simulink model "Copy_of_minimal_rcu_full"  (R2014b)
settings: Solver=ode4  SolverMode=SingleTasking  StartTime=0.0  StopTime=t_sim  FixedStep=sample_time_model  RelTol=1e-3
PreLoadFcn:
  | initModell
InitFcn:
  | initModell
undefined symbols (not defined in the file): FILTER_TAU_EXT, FIXED_FILTER_BANDWIDTH, FIXED_FILTER_BANDWIDTH_OBSERVER, iter, K_INV, KI2TAU_VEC, KS_trq, KT_trq, load_inertia, load_mass, MAX_CURRENT, MIN_SING_VALUE_M_CART, q0, rCEE_i, sample_time_model, sample_time_robot, tau_max
libraries: simulink x69, robotics x15, beasty_sfcns x7, lwr_dynamics x6, trafo3dLib x4, holgersRobLib x3, dspmtrx3 x1, dspinverses x1
(part 1 of 4)
settings Model: ExtModeAutoUpdateStatusClock=off  Creator=krie_ka  LastModifiedBy=lilge
settings DataIOCC: ExternalInput=[t u]  SignalLoggingSaveFormat=ModelDataLogs
settings OptimizationCC: ExpressionDepthLimit=2147483647  InitFltsAndDblsToZero=on
settings DebuggingCC: SaveWithParameterizedLinksMsg=none  UnderspecifiedInitializationDetection=Classic  MergeDetectMultiDrivingBlocksExec=none  FcnCallInpInsideContextMsg=UseLocalSettings  StateNameClashWarn=warning
settings HardwareCC: TargetHWDeviceType=32-bit Generic
settings SFSimCC: SimParseCustomCode=off
settings GRTTargetCC: TargetFcnLib=ansi_tfl_tmw.mat  CombineOutputUpdateFcns=off  GRTInterface=on

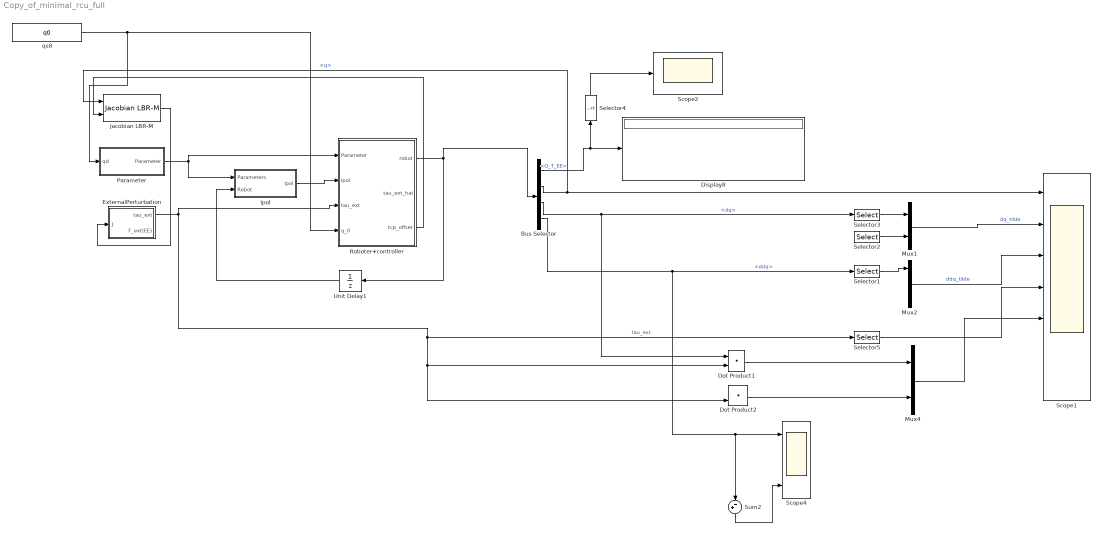
== system Copy_of_minimal_rcu_full ==
  Bus Selector : BusSelector  OutputSignals=Transform_theta.O_T_EE,q,dq,ddq
  Display8 : Display
  Dot Product1 : DotProduct  InputSameDT=on  OutDataTypeStr=Inherit: Inherit via internal rule
  Dot Product2 : DotProduct  InputSameDT=on  OutDataTypeStr=Inherit: Inherit via internal rule
  ExternalPerturbation : Subsystem
  Ipol : Subsystem
  Jacobian LBR-M : holgersRobLib/Jacobian LBR-M
  Mux1 : Mux  Inputs=2
  Mux2 : Mux  Inputs=3
  Mux4 : Mux  Inputs=2
  Parameter : Subsystem
  Roboter+controller : Subsystem
  Scope1 : Scope  NumInputPorts=7
      settings: TimeRange=1  YMin=-2~-0.04~-40~-1~-1~-1~-1  YMax=1~0.04~20~1~1~1~1  SaveName=ScopeData4
  Scope2 : Scope
      settings: TimeRange=1.4  YMin=-0.6  YMax=0.8  SaveName=ScopeData5
  Scope4 : Scope  NumInputPorts=3
      settings: TimeRange=0.06  YMin=-60~-60~-60  YMax=80~60~60  SaveName=ScopeData7
  Selector1 : Selector  InputPortWidth=7  Indices=[1:7]
  Selector2 : Selector  InputPortWidth=7  Indices=[6,7]
  Selector3 : Selector  InputPortWidth=7  Indices=[6,7]
  Selector4 : Selector  NumberOfDimensions=2  InputPortWidth=7  IndexOptions=Index vector (dialog),Index vector (dialog)  Indices=1:3,4  OutputSizes=1,1
  Selector5 : Selector  InputPortWidth=7  Indices=7
  Sum2 : Sum  Inputs=+-|
  Unit Delay1 : UnitDelay  SampleTime=-1
  qs8 : Constant  Value=q0
  wires:
  Parameter/1(Parameter) -> Roboter+controller/1(Parameter), Ipol/1(Parameters)
  Ipol/1(ipol) -> Roboter+controller/2(ipol)
  Unit Delay1/1 -> Ipol/2(Robot)
  Roboter+controller/1(robot) -> Unit Delay1/1, Bus Selector/1
  Bus Selector/3 -> Dot Product1/1, Selector3/1  "<dq>"
  Mux2/1 -> Scope1/3  "ddq_tilde"
  Bus Selector/2 -> Scope1/1, Jacobian LBR-M/1  "<q>"
  Bus Selector/1 -> Display8/1, Selector4/1  "<O_T_EE>"
  Selector1/1 -> Mux2/1
  Mux1/1 -> Scope1/2  "dq_tilde"
  Selector2/1 -> Mux1/2
  Selector3/1 -> Mux1/1
  Selector4/1 -> Scope2/1
  qs8/1 -> Parameter/1(qd), Roboter+controller/4(q_0)
  ExternalPerturbation/1(tau_ext) -> Roboter+controller/3(tau_ext), Dot Product2/2, Dot Product1/2, Selector5/1  "tau_ext"
  Selector5/1 -> Scope1/4
  Dot Product1/1 -> Mux4/1
  Dot Product2/1 -> Mux4/2
  Mux4/1 -> Scope1/5
  Jacobian LBR-M/1 -> ExternalPerturbation/1(J)
  Sum2/1 -> Scope4/3
  Bus Selector/4 -> Scope4/1, Sum2/2, Selector1/1  "<ddq>"
  Roboter+controller/3(tcp_offset) -> Jacobian LBR-M/2

== system Copy_of_minimal_rcu_full/ExternalPerturbation ==
  J : Inport
  F_ext (EE) : Constant  Tag=Fext  Value=[0; 0; 0; 0; 0; 0]
  Product : Product  Multiplication=Matrix(*)  RndMeth=Zero
  Transpose : dspmtrx3/Transpose  Hermitian=off  overflowFlag=off
  tau_ext : Outport
  F_ext(EE) : Outport  Port=2
  wires:
  Product/1 -> tau_ext/1
  J/1 -> Transpose/1
  Transpose/1 -> Product/1
  F_ext (EE)/1 -> F_ext(EE)/1, Product/2

== system Copy_of_minimal_rcu_full/Ipol ==
  Parameters : Inport
  Robot : Inport  Port=2
  Bus Creator : BusCreator  Inputs=6
  Bus Creator1 : BusCreator  Inputs=6
  Manual Switch : ManualSwitch  CurrentSetting=0
  custom : Subsystem
  dq_max1 : Constant  Value=zeros(7,1)
  dq_max5 : Constant  Value=zeros(7,1)
  dq_max6 : Constant
  dq_max7 : Constant  Value=0
  joint_ipol_5th_traj_scaling : Subsystem
  ipol : Outport
  wires:
  Parameters/1 -> custom/1(parameters), joint_ipol_5th_traj_scaling/1(parameters)
  Robot/1 -> joint_ipol_5th_traj_scaling/2(robot)
  joint_ipol_5th_traj_scaling/1(q_d) -> Bus Creator/1  "theta_d"
  joint_ipol_5th_traj_scaling/2(dq_d) -> Bus Creator/2  "dtheta_d"
  joint_ipol_5th_traj_scaling/3(ddq_d) -> Bus Creator/3  "ddtheta_d"
  joint_ipol_5th_traj_scaling/4(T_d) -> Bus Creator/4  "0_T_EE_d"
  joint_ipol_5th_traj_scaling/5(0_dX_d) -> Bus Creator/5  "0_dx_d"
  dq_max5/1 -> Bus Creator/6  "0_ddx_d"
  Bus Creator/1 -> Manual Switch/1
  dq_max6/1 -> joint_ipol_5th_traj_scaling/4(enable), joint_ipol_5th_traj_scaling/3(start1)
  dq_max7/1 -> joint_ipol_5th_traj_scaling/5(reset)
  custom/1(q_d) -> Bus Creator1/1  "theta_d"
  custom/2(dq_d) -> Bus Creator1/2  "dtheta_d"
  custom/3(ddq_d) -> Bus Creator1/3  "ddtheta_d"
  custom/4(T_d) -> Bus Creator1/4  "0_T_EE_d"
  custom/5(0_dX_d) -> Bus Creator1/5  "0_dx_d"
  dq_max1/1 -> Bus Creator1/6  "0_ddx_d"
  Bus Creator1/1 -> Manual Switch/2
  Manual Switch/1 -> ipol/1

== system Copy_of_minimal_rcu_full/Parameter ==
  qd : Inport
  Bus Creator : BusCreator  Inputs=25
  control : Subsystem
  ipol : Subsystem
  load : Subsystem
  Parameter : Outport
  wires:
  load/3(I_EE_) -> Bus Creator/3  "I_EE"
  Bus Creator/1 -> Parameter/1
  load/4(g_) -> Bus Creator/4  "g"
  control/1(controller) -> Bus Creator/5  "controller"
  control/2(enable_ffwd_vel_) -> Bus Creator/6  "enable_ffwd_vel"
  control/3(enable_ffwd_acc_) -> Bus Creator/7  "enable_ffwd_acc"
  control/4(K_theta_) -> Bus Creator/8  "K_theta"
  control/5(D_theta_) -> Bus Creator/9  "D_theta"
  control/6(TCP_T_EE_) -> Bus Creator/10  "TCP_T_EE"
  control/7(W_T_O_) -> Bus Creator/11  "W_T_0"
  control/8(EE_T_K_) -> Bus Creator/12  "EE_T_K"
  control/9(K_x_) -> Bus Creator/13  "K_x"
  control/10(D_x_) -> Bus Creator/14  "D_x"
  control/11(K_NS_) -> Bus Creator/15  "K_NS"
  control/12(Xi_NS_) -> Bus Creator/16  "Xi_NS"
  control/13(W_NS_dir_) -> Bus Creator/17  "W_NS_dir"
  load/1(m_EE_) -> Bus Creator/1  "mEE"
  load/2(rC_EE_) -> Bus Creator/2  "rC_EE"
  ipol/1(ipol_type) -> Bus Creator/18  "ipol_type"
  ipol/2(enable1) -> Bus Creator/19  "ipol_start"
  ipol/3(q2_) -> Bus Creator/20  "q2"
  ipol/4(dq_max_) -> Bus Creator/21  "dq_max"
  ipol/5(ddqd_max_) -> Bus Creator/22  "ddq_max"
  ipol/6(O_T_2_) -> Bus Creator/23  "0_T_2"
  ipol/7(O_T_d_In_) -> Bus Creator/24  "0_T_d_In"
  ipol/8(dX_max_) -> Bus Creator/25  "dX_max"
  qd/1 -> ipol/1(q2)

== system Copy_of_minimal_rcu_full/Roboter+controller ==
  Parameter : Inport
  ipol : Inport  Port=2
  tau_ext : Inport  Port=3
  q_0 : Inport  Port=4
  State_Observer : Subsystem
  controller : Subsystem
  force esimation : Subsystem
  robot_simulation : Subsystem
  robot : Outport
  tau_ext_hat : Outport  Port=2
  tcp_offset : Outport  Port=3
  wires:
  controller/1(gains) -> robot_simulation/2(gains)
  robot_simulation/1(robot) -> robot/1, force esimation/1(Robot), controller/3(robot), State_Observer/1(robot_model)
  Parameter/1 -> controller/1(parameters), robot_simulation/1(parameters)
  controller/2(tau_d) -> robot_simulation/3(tau)
  ipol/1 -> controller/2(ipol)
  State_Observer/1(r_filtered) -> tau_ext_hat/1
  tau_ext/1 -> robot_simulation/4(tau_ext)
  q_0/1 -> robot_simulation/5(q_0)
  controller/3(tcp_offset) -> tcp_offset/1
  robot_simulation/2(w/o load) -> State_Observer/2(robot_model1)
  State_Observer/2(r_filtered1) -> force esimation/2(tau_ext)

== system Copy_of_minimal_rcu_full/Ipol/custom ==
  parameters : Inport
  Bus Selector3 : BusSelector  OutputSignals=q2,dq_max,ddq_max,TCP_T_EE
  Calc Fkin2 : Subsystem  SystemSampleTime=0.034
  Clock : Clock
  Discrete Derivative1 : simulink/Discrete/Discrete Derivative  gainval=1.0  ICPrevScaledInput=0.0  InputProcessing=Inherited  OutMin=[]  OutMax=[]  OutDataType=sfix(16)  OutScaling=2^-10  DoSatur=off
  Discrete Derivative2 : simulink/Discrete/Discrete Derivative  gainval=1.0  ICPrevScaledInput=0.0  InputProcessing=Inherited  OutMin=[]  OutMax=[]  OutDataType=sfix(16)  OutScaling=2^-10  DoSatur=off
  Mux3 : Mux  Inputs=1
  Reshape1 : Reshape  OutputDimensions=[3,4]
  Reshape4 : Reshape  OutputDimensions=[3,4]
  Selector : Selector  NumberOfDimensions=2  InputPortWidth=3  IndexOptions=Index vector (dialog),Index vector (dialog)  Indices=[1:3],4  OutputSizes=1,1
  Sine Wave Function : Sin  Amplitude=0.0  Frequency=3  SampleTime=0
  Trigonometric Function : Trigonometry
  qs1 : Constant  Value=q0
  qs2 : Constant  Value=q0
  q_d : Outport
  dq_d : Outport  Port=2
  ddq_d : Outport  Port=3
  T_d : Outport  Port=4
  0_dX_d : Outport  Port=5
  wires:
  Calc Fkin2/1(FKin_d2) -> Reshape4/1, Selector/1
  Mux3/1 -> Discrete Derivative2/1, q_d/1, Calc Fkin2/1(In1)
  Selector/1 -> Discrete Derivative1/1
  Discrete Derivative1/1 -> Reshape1/1  "O_dX_d"
  Reshape1/1 -> 0_dX_d/1  "O_dX_d"
  Discrete Derivative2/1 -> dq_d/1
  qs1/1 -> Mux3/1
  Clock/1 -> Trigonometric Function/1
  Trigonometric Function/1 -> ?
  parameters/1 -> Bus Selector3/1
  Bus Selector3/4 -> Calc Fkin2/2(TCP_T_EE)  "<TCP_T_EE>"
  qs2/1 -> ddq_d/1
  Reshape4/1 -> T_d/1  "T_d"

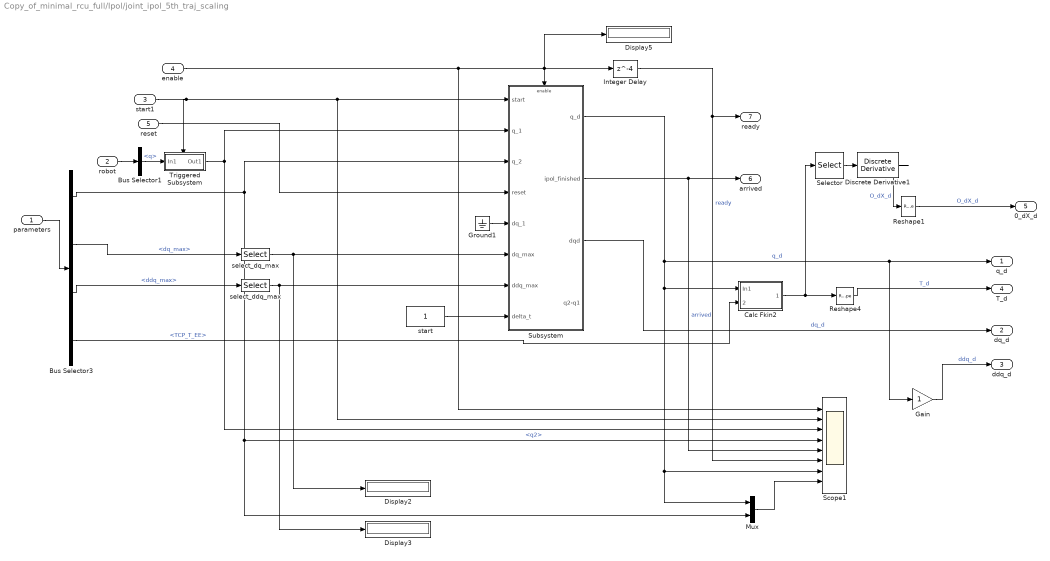
== system Copy_of_minimal_rcu_full/Ipol/joint_ipol_5th_traj_scaling ==
  parameters : Inport
  robot : Inport  Port=2
  start1 : Inport  Port=3
  enable : Inport  Port=4
  reset : Inport  Port=5
  Bus Selector1 : BusSelector  OutputSignals=q
  Bus Selector3 : BusSelector  OutputSignals=q2,dq_max,ddq_max,TCP_T_EE
  Calc Fkin2 : Subsystem  SystemSampleTime=0.034
  Discrete Derivative1 : simulink/Discrete/Discrete Derivative  gainval=1.0  ICPrevScaledInput=0.0  InputProcessing=Inherited  OutMin=[]  OutMax=[]  OutDataType=sfix(16)  OutScaling=2^-10  DoSatur=off
  Display2 : Display
  Display3 : Display
  Display5 : Display
  Gain : Gain
  Ground1 : Ground
  Integer Delay : Delay  DelayLength=4  InputProcessing=Inherited
  Mux : Mux  Inputs=2
  Reshape1 : Reshape  OutputDimensions=[3,4]
  Reshape4 : Reshape  OutputDimensions=[3,4]
  Scope1 : Scope  NumInputPorts=8
      settings: YMin=-1~-1~-0.1~0~0.95~-1~0~0  YMax=1~1~0.8~1~1.05~1~1~1  SaveName=ScopeData52
  Selector : Selector  NumberOfDimensions=2  InputPortWidth=3  IndexOptions=Index vector (dialog),Index vector (dialog)  Indices=[1:3],4  OutputSizes=1,1
  Subsystem : Subsystem
  Triggered Subsystem : Subsystem  TreatAsAtomicUnit=on
  select_ddq_max : Selector  InputPortWidth=7  Indices=[1]
  select_dq_max : Selector  InputPortWidth=7  Indices=[1]
  start : Constant
  q_d : Outport
  dq_d : Outport  Port=2
  ddq_d : Outport  Port=3
  T_d : Outport  Port=4
  0_dX_d : Outport  Port=5
  arrived : Outport  Port=6
  ready : Outport  Port=7
  wires:
  Bus Selector3/3 -> select_ddq_max/1  "<ddq_max>"
  Bus Selector3/2 -> select_dq_max/1  "<dq_max>"
  Reshape1/1 -> 0_dX_d/1  "O_dX_d"
  Discrete Derivative1/1 -> Reshape1/1  "O_dX_d"
  Selector/1 -> Discrete Derivative1/1
  Subsystem/3(dqd) -> dq_d/1  "dq_d"
  Subsystem/1(q_d) -> Calc Fkin2/1(In1), Mux/1, Scope1/7, Gain/1, q_d/1  "q_d"
  Ground1/1 -> Subsystem/5(dq_1)
  Mux/1 -> Scope1/8
  Reshape4/1 -> T_d/1  "T_d"
  Calc Fkin2/1(FKin_d2) -> Selector/1, Reshape4/1
  Subsystem/2(ipol_finished) -> Scope1/5, arrived/1  "arrived"
  parameters/1 -> Bus Selector3/1
  Integer Delay/1 -> Scope1/6, ready/1  "ready"
  Triggered Subsystem/1(Out1) -> Scope1/3, Subsystem/2(q_1)
  Bus Selector3/1 -> Mux/2, Scope1/4, Subsystem/3(q_2)  "<q2>"
  select_dq_max/1 -> Display2/1, Subsystem/6(dq_max)
  select_ddq_max/1 -> Display3/1, Subsystem/7(ddq_max)
  Gain/1 -> ddq_d/1  "ddq_d"
  robot/1 -> Bus Selector1/1
  Bus Selector1/1 -> Triggered Subsystem/1(In1)  "<q>"
  enable/1 -> Subsystem/Enable, Integer Delay/1, Display5/1, Scope1/1
  start/1 -> Subsystem/8(delta_t)
  start1/1 -> Scope1/2, Subsystem/1(start), Triggered Subsystem/Trigger
  reset/1 -> Subsystem/4(reset)
  Bus Selector3/4 -> Calc Fkin2/2(TCP_T_EE)  "<TCP_T_EE>"

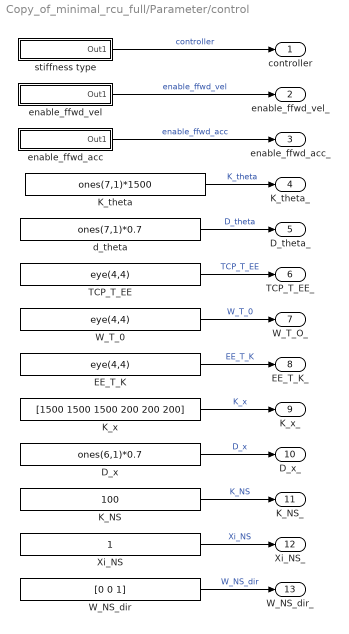
== system Copy_of_minimal_rcu_full/Parameter/control ==
  D_x : Constant  Value=ones(6,1)*0.7
  EE_T_K : Constant  Value=eye(4,4)
  K_NS : Constant  Value=100
  K_theta : Constant  Value=ones(7,1)*1500
  K_x : Constant  Value=[1500 1500 1500 200 200 200]
  TCP_T_EE : Constant  Value=eye(4,4)
  W_NS_dir : Constant  Value=[0 0 1]
  W_T_0 : Constant  Value=eye(4,4)
  Xi_NS : Constant
  d_theta : Constant  Value=ones(7,1)*0.7
  enable_ffwd_acc : Subsystem  mask{controller_type=off}
      mask prompts: controller_type "Enable"
      mask init:
      | ctrlp(1).s='false';
      | ctrlp(2).s='true';
      mask Display: fprintf('Ctrl = %s', ctrlp(controller_type+1).s)
  enable_ffwd_vel : Subsystem  mask{controller_type=off}
      mask prompts: controller_type "Enable"
      mask init:
      | ctrlp(1).s='false';
      | ctrlp(2).s='true';
      mask Display: fprintf('Ctrl = %s', ctrlp(controller_type+1).s)
  stiffness type : Subsystem  mask{controller_type=2 ... Joint Impedance}
      mask prompts: controller_type "Type"
      mask init:
      | ctrlp(1).s='cart';
      | ctrlp(2).s='joint';
      mask TypeOptions controller_type: 1 ... Cartesian Impedance | 2 ... Joint Impedance
      mask Display: fprintf('Ctrl = %s', ctrlp(controller_type).s)
  controller : Outport
  enable_ffwd_vel_ : Outport  Port=2
  enable_ffwd_acc_ : Outport  Port=3
  K_theta_ : Outport  Port=4
  D_theta_ : Outport  Port=5
  TCP_T_EE_ : Outport  Port=6
  W_T_O_ : Outport  Port=7
  EE_T_K_ : Outport  Port=8
  K_x_ : Outport  Port=9
  D_x_ : Outport  Port=10
  K_NS_ : Outport  Port=11
  Xi_NS_ : Outport  Port=12
  W_NS_dir_ : Outport  Port=13
  wires:
  stiffness type/1(Out1) -> controller/1  "controller"
  enable_ffwd_vel/1(Out1) -> enable_ffwd_vel_/1  "enable_ffwd_vel"
  enable_ffwd_acc/1(Out1) -> enable_ffwd_acc_/1  "enable_ffwd_acc"
  K_theta/1 -> K_theta_/1  "K_theta"
  d_theta/1 -> D_theta_/1  "D_theta"
  TCP_T_EE/1 -> TCP_T_EE_/1  "TCP_T_EE"
  W_T_0/1 -> W_T_O_/1  "W_T_0"
  EE_T_K/1 -> EE_T_K_/1  "EE_T_K"
  K_x/1 -> K_x_/1  "K_x"
  D_x/1 -> D_x_/1  "D_x"
  K_NS/1 -> K_NS_/1  "K_NS"
  Xi_NS/1 -> Xi_NS_/1  "Xi_NS"
  W_NS_dir/1 -> W_NS_dir_/1  "W_NS_dir"

== system Copy_of_minimal_rcu_full/Parameter/ipol ==
  q2 : Inport
  0 : Constant  Value=0
  1 : Constant
  Manual Switch : ManualSwitch  CurrentSetting=0
  Manual Switch1 : ManualSwitch
  O_T_1 : Constant  Value=[1 0 0 0 0 1 0 -1 0 0.3 -0.3 0.7]
  O_T_2 : Constant  Value=[1 0 0 0 1 0 0 0 1 0.3 0.3 0.7]
  O_T_d_In : Constant  Value=[1 0 0 0 1 0 0 0 1 -0.3 -0.3 0.7]
  dX_max : Constant  Value=ones(6,1)*1
  ddqd_max : Constant  Value=ones(7,1)
  dq_max : Constant  Value=ones(7,1)
  stiffness type : Subsystem  mask{controller_type=2 ... joint 5th scaling}
      mask prompts: controller_type "Type"
      mask init:
      | ctrlp(2).s='joint 5th';
      | ctrlp(1).s='cart attra';
      mask TypeOptions controller_type: 1 ... cart attractor | 2 ... joint 5th scaling
      mask Display: fprintf('Ctrl = %s', ctrlp(controller_type).s)
  ipol_type : Outport
  enable1 : Outport  Port=2
  q2_ : Outport  Port=3
  dq_max_ : Outport  Port=4
  ddqd_max_ : Outport  Port=5
  O_T_2_ : Outport  Port=6
  O_T_d_In_ : Outport  Port=7
  dX_max_ : Outport  Port=8
  wires:
  dq_max/1 -> dq_max_/1
  ddqd_max/1 -> ddqd_max_/1
  O_T_d_In/1 -> O_T_d_In_/1
  dX_max/1 -> dX_max_/1
  stiffness type/1(Out1) -> ipol_type/1
  Manual Switch1/1 -> enable1/1
  O_T_2/1 -> Manual Switch/1
  O_T_1/1 -> Manual Switch/2
  Manual Switch/1 -> O_T_2_/1
  0/1 -> Manual Switch1/1
  1/1 -> Manual Switch1/2
  q2/1 -> q2_/1

== system Copy_of_minimal_rcu_full/Parameter/load ==
  Display8 : Display
  Product : Product  Inputs=3  RndMeth=Zero
  g : Constant  Value=[0 0 9.81]
  m_EE : Constant
  rCEE : Constant  Value=rCEE_i
  m_EE_ : Outport
  rC_EE_ : Outport  Port=2
  I_EE_ : Outport  Port=3
  g_ : Outport  Port=4
  wires:
  rCEE/1 -> Product/2, Product/3, Display8/1, rC_EE_/1  "rC_EE"
  m_EE/1 -> Product/1, m_EE_/1  "m_EE"
  Product/1 -> I_EE_/1  "I_EE"
  g/1 -> g_/1  "g"

== system Copy_of_minimal_rcu_full/Roboter+controller/State_Observer ==
  robot_model : Inport
  robot_model1 : Inport  Port=2
  Bus Selector1 : BusSelector  OutputSignals=dq,tau_a,dynamics_q.G,dynamics_q.C,dynamics_q.Mass
  Bus Selector2 : BusSelector  OutputSignals=Mass1,C1,G1,m_EE1,I_EE
  Constant7 : Constant  Value=[0 0 0 0 0 0 0]
  First_order_filter1 : Subsystem  mask{h=sample_time_robot, T=1./( 2*pi *FILTER_TAU_EXT)}
      mask help:
      | c1 = h/(h+T)
      | c2 = T/(h+T)
      | h - sampling time
      | T =1/(2*pi*f) filter time constant
      | y[n] = c1*x[n] + c2*y[n-1]
  Impulse_Observer : Subsystem
  K1_beo1 : Constant
  Reshape1 : Reshape  OutputDimensionality=Customize  OutputDimensions=[7,7]
  Terminator{2..7} (6 alike) : Terminator
  reset : Constant  Value=0
  r_filtered : Outport
  r_filtered1 : Outport  Port=2
  wires:
  Constant7/1 -> First_order_filter1/2(d_delta_p)
  K1_beo1/1 -> Impulse_Observer/6(K1_beo)
  Impulse_Observer/1(r) -> First_order_filter1/1(x[n])
  Impulse_Observer/3(p) -> Terminator2/1
  Impulse_Observer/4(p_hat) -> Terminator3/1
  Impulse_Observer/8(n) -> Terminator7/1
  Impulse_Observer/5(beta) -> Terminator4/1
  Impulse_Observer/7(dMq) -> Terminator6/1
  Impulse_Observer/6(dM) -> Terminator5/1
  robot_model/1 -> Bus Selector1/1
  Reshape1/1 -> Impulse_Observer/5(M)
  First_order_filter1/1(y[n]) -> r_filtered/1
  reset/1 -> First_order_filter1/3(reset), Impulse_Observer/7(reset)
  robot_model1/1 -> Bus Selector2/1
  Bus Selector2/1 -> Reshape1/1  "<Mass1>"
  Bus Selector2/2 -> Impulse_Observer/4(C)  "<C1>"
  Bus Selector2/3 -> Impulse_Observer/3(G)  "<G1>"
  Bus Selector1/1 -> Impulse_Observer/1(dq)  "<dq>"
  Bus Selector1/2 -> Impulse_Observer/2(tau)  "<tau_a>"
  Impulse_Observer/2(r_unfiltered) -> r_filtered1/1

== system Copy_of_minimal_rcu_full/Roboter+controller/controller ==
  parameters : Inport
  ipol : Inport  Port=2
  robot : Inport  Port=3
  Bus Selector : BusSelector  OutputSignals=controller
  Cartesian Impedance Control : Subsystem
  Index Vector : MultiPortSwitch  Inputs=2
  Joint Impedance : Subsystem
  gains_selector : Subsystem
  gains : Outport
  tau_d : Outport  Port=2
  tcp_offset : Outport  Port=3
  wires:
  gains_selector/1(gains) -> gains/1
  Bus Selector/1 -> gains_selector/1(controller), Index Vector/1  "<controller>"
  parameters/1 -> Bus Selector/1, Joint Impedance/2(parameters), Cartesian Impedance Control/2(Parameter)
  gains_selector/2(B_theta) -> Joint Impedance/1(B_theta), Cartesian Impedance Control/1(B_theta)
  robot/1 -> Joint Impedance/3(robot), Cartesian Impedance Control/3(robot)
  ipol/1 -> Joint Impedance/4(ipol), Cartesian Impedance Control/4(IPOL)
  Index Vector/1 -> tau_d/1
  Cartesian Impedance Control/1(cart_imp) -> Index Vector/2
  Joint Impedance/1(tau_d) -> Index Vector/3
  Cartesian Impedance Control/2(tcp_offset) -> tcp_offset/1

== system Copy_of_minimal_rcu_full/Roboter+controller/force esimation ==
  Robot : Inport
  tau_ext : Inport  Port=2
  " LU Inverse" : dspinverses/ LU Inverse
  Bus Selector : BusSelector  OutputSignals=body_jacobians.B_JT_6,zero_jacobians.O_JT_6
  Product : Product  Multiplication=Matrix(*)  RndMeth=Zero
  Reshape5 : Reshape  OutputDimensionality=Customize  OutputDimensions=[7,6]
  Scope1 : Scope
      settings: TimeRange=1  YMin=-8  YMax=4  SaveName=ScopeData6
  Scope3 : Scope
      settings: TimeRange=10  YMin=-2  YMax=12  SaveName=ScopeData2
  Selector1 : Selector  NumberOfDimensions=2  InputPortWidth=7  IndexOptions=Index vector (dialog),Index vector (dialog)  Indices=[1:6],[1:6]  OutputSizes=1,1
  Selector2 : Selector  InputPortWidth=7  Indices=[1:6]
  To Workspace : ToWorkspace  VariableName=F_ext_6  SaveFormat=Structure  SampleTime=-1
  To Workspace1 : ToWorkspace  VariableName=tau_ext_hat  SaveFormat=Structure  SampleTime=-1
  wires:
  Robot/1 -> Bus Selector/1
  Product/1 -> To Workspace/1, Scope3/1
  " LU Inverse"/1 -> Product/1
  Reshape5/1 -> Selector1/1
  tau_ext/1 -> Selector2/1, To Workspace1/1, Scope1/1
  Selector2/1 -> Product/2
  Selector1/1 -> " LU Inverse"/1
  Bus Selector/2 -> Reshape5/1  "<O_JT_6>"

== system Copy_of_minimal_rcu_full/Roboter+controller/robot_simulation ==
  parameters : Inport
  gains : Inport  Port=2
  tau : Inport  Port=3
  tau_ext : Inport  Port=4
  q_0 : Inport  Port=5
  Bus Creator4 : BusCreator  Inputs=11
  Bus Selector1 : BusSelector  OutputSignals=TCP_T_EE
  Bus Selector3 : BusSelector  OutputSignals=mEE,rC_EE,I_EE,g
  Dynamics : Subsystem
  Sum : Sum  Inputs=|++
  model : Subsystem
  robot : Outport
  w/o load : Outport  Port=2
  wires:
  Bus Selector3/1 -> Dynamics/1(m_EE)  "<mEE>"
  Bus Selector3/2 -> Dynamics/2(rC_EE)  "<rC_EE>"
  Bus Selector3/3 -> Dynamics/3(I_EE)  "<I_EE>"
  Bus Selector3/4 -> Dynamics/4(g)  "<g>"
  parameters/1 -> Bus Selector3/1, [parameter]
  gains/1 -> Dynamics/6(Gains)
  Dynamics/1(q) -> model/1(q), Bus Creator4/5  "q"
  Dynamics/2(dq) -> Bus Creator4/6  "dq"
  model/1(body_jacobians) -> Bus Creator4/1  "body_jacobians"
  model/2(zero_jacobians) -> Bus Creator4/2  "zero_jacobians"
  model/3(Transforms_q) -> Bus Creator4/3  "Transform_q"
  Dynamics/3(theta) -> Bus Creator4/7, model/3(theta)  "theta"
  Dynamics/4(dtheta) -> Bus Creator4/8  "dtheta"
  Bus Creator4/1 -> robot/1
  Dynamics/5(dynamics_q) -> Bus Creator4/9  "dynamics_q"
  Bus Selector1/1 -> model/2(TCP_T_EE)  "<TCP_T_EE>"
  [parameter] -> Bus Selector1/1
  model/4(Transforms_theta) -> Bus Creator4/4  "Transform_theta"
  tau_ext/1 -> Dynamics/7(tau_ext)
  Dynamics/6(tau) -> Bus Creator4/10
  q_0/1 -> Dynamics/8(q_0)
  tau/1 -> Sum/1
  Sum/1 -> Dynamics/5(tau_d)
  Dynamics/7(dyn_w/o_load) -> w/o load/1
  Dynamics/8(ddq) -> Bus Creator4/11  "ddq"

== system Copy_of_minimal_rcu_full/Ipol/custom/Calc Fkin2 ==
  In1 : Inport
  TCP_T_EE : Inport  Port=2
  Forward Kinematics LBR-M3 : S-Function  FunctionName=lbrmdirkin_sfun  EnableBusSupport=off
      mask help:
      | lbrMDirKin_sfun
      | Last update: 17.03.2008
      |
      | Input 1: Position (7)
      | Input 2: TCP trafo   (3x4)
      mask Help:
      | HELP for S-Function lbrMDirKinSfun:<br>
      | ===========================<br>
      | <br>
      | Input Arguments [1]:<br>
      | --------------<br>
      | u = q<br>
      | <br>
      | Output Arguments [1]:<br>
      | ---------------<br>
      | y = TCP-Frame ... as a 3x4-matrix<br>
      mask Display: disp('LBR-M\nKinematics')
  Reshape4 : Reshape  OutputDimensionality=Customize  OutputDimensions=[4,4]
  Selector1 : Selector  NumberOfDimensions=2  InputPortWidth=3  IndexOptions=Index vector (dialog),Select all  Indices=1:3,-1
  FKin_d2 : Outport
  wires:
  Selector1/1 -> Forward Kinematics LBR-M3/2
  In1/1 -> Forward Kinematics LBR-M3/1
  Forward Kinematics LBR-M3/1 -> FKin_d2/1
  Reshape4/1 -> Selector1/1
  TCP_T_EE/1 -> Reshape4/1

== system Copy_of_minimal_rcu_full/Ipol/joint_ipol_5th_traj_scaling/Calc Fkin2 ==
  In1 : Inport
  TCP_T_EE : Inport  Port=2
  Forward Kinematics LBR-M3 : S-Function  FunctionName=lbrmdirkin_sfun  EnableBusSupport=off
      mask help:
      | lbrMDirKin_sfun
      | Last update: 17.03.2008
      |
      | Input 1: Position (7)
      | Input 2: TCP trafo   (3x4)
      mask Help:
      | HELP for S-Function lbrMDirKinSfun:<br>
      | ===========================<br>
      | <br>
      | Input Arguments [1]:<br>
      | --------------<br>
      | u = q<br>
      | <br>
      | Output Arguments [1]:<br>
      | ---------------<br>
      | y = TCP-Frame ... as a 3x4-matrix<br>
      mask Display: disp('LBR-M\nKinematics')
  Reshape4 : Reshape  OutputDimensionality=Customize  OutputDimensions=[4,4]
  Selector1 : Selector  NumberOfDimensions=2  InputPortWidth=3  IndexOptions=Index vector (dialog),Select all  Indices=1:3,-1
  FKin_d2 : Outport
  wires:
  TCP_T_EE/1 -> Reshape4/1
  Reshape4/1 -> Selector1/1
  Forward Kinematics LBR-M3/1 -> FKin_d2/1
  In1/1 -> Forward Kinematics LBR-M3/1
  Selector1/1 -> Forward Kinematics LBR-M3/2

== system Copy_of_minimal_rcu_full/Ipol/joint_ipol_5th_traj_scaling/Subsystem ==
  start : Inport
  q_1 : Inport  Port=2
  q_2 : Inport  Port=3
  reset : Inport  Port=4
  dq_1 : Inport  Port=5
  dq_max : Inport  Port=6
  ddq_max : Inport  Port=7
  delta_t : Inport  Port=8
  Enable : EnablePort
  Add : Sum  Inputs=+-
  Cartesian_ipol1 : Subsystem  TreatAsAtomicUnit=on
  Compare To Zero : simulink/Logic and Bit Operations/Compare To Zero  relop=>  OutDataTypeStr=uint8  ZeroCross=off
  Data Type Conversion1 : DataTypeConversion  OutDataTypeStr=double
  Detect Increase1 : simulink/Logic and Bit Operations/Detect Increase  vinit=0.0  InputProcessing=Inherited  OutDataTypeStr=uint8
  Detect Increase2 : simulink/Logic and Bit Operations/Detect Increase  vinit=0.0  InputProcessing=Inherited  OutDataTypeStr=uint8
  Detect Increase3 : simulink/Logic and Bit Operations/Detect Increase  vinit=0.0  InputProcessing=Inherited  OutDataTypeStr=uint8
  Digital Clock2 : DigitalClock  SampleTime=sample_time_model
  Logical Operator : Logic  Operator=OR  Inputs=3  AllPortsSameDT=off  OutDataTypeStr=boolean
  Logical Operator1 : Logic  Operator=OR  AllPortsSameDT=off  OutDataTypeStr=boolean
  Logical Operator3 : Logic  Operator=OR  AllPortsSameDT=off  OutDataTypeStr=boolean
  Unit Delay1 : UnitDelay  SampleTime=-1
  time_generator and resets : Subsystem
  q_d : Outport
  ipol_finished : Outport  Port=2
  dqd : Outport  Port=3
  q2-q1 : Outport  Port=4
  wires:
  Add/1 -> q2-q1/1
  Cartesian_ipol1/3(dqd) -> dqd/1
  delta_t/1 -> time_generator and resets/3(delta_t)
  dq_1/1 -> Cartesian_ipol1/3(v0)
  Cartesian_ipol1/2(ipol_finished) -> ipol_finished/1
  Cartesian_ipol1/1(qd) -> q_d/1
  reset/1 -> Detect Increase1/1
  q_2/1 -> Add/1, Cartesian_ipol1/4(sf)
  q_1/1 -> Add/2, Cartesian_ipol1/2(s0)
  start/1 -> Logical Operator/2, time_generator and resets/1(start), Detect Increase3/1
  ddq_max/1 -> Cartesian_ipol1/6(am)
  dq_max/1 -> Cartesian_ipol1/5(vm)
  Logical Operator3/1 -> time_generator and resets/2(reset)
  Data Type Conversion1/1 -> Logical Operator3/1, Logical Operator/3
  Digital Clock2/1 -> Compare To Zero/1
  Compare To Zero/1 -> Detect Increase2/1
  Logical Operator/1 -> Cartesian_ipol1/Enable
  time_generator and resets/1(time) -> Cartesian_ipol1/1(t)
  Detect Increase2/1 -> Unit Delay1/1, Logical Operator3/2
  Logical Operator1/1 -> Data Type Conversion1/1
  Detect Increase1/1 -> Logical Operator1/2
  Detect Increase3/1 -> Logical Operator1/1
  Unit Delay1/1 -> Logical Operator/1

== system Copy_of_minimal_rcu_full/Ipol/joint_ipol_5th_traj_scaling/Triggered Subsystem ==
  In1 : Inport
  Trigger : TriggerPort
  Out1 : Outport
  wires:
  In1/1 -> Out1/1

== system Copy_of_minimal_rcu_full/Parameter/control/enable_ffwd_acc ==
  Controller type : Constant  Value=controller_type  OutDataTypeStr=double
  Out1 : Outport
  wires:
  Controller type/1 -> Out1/1

== system Copy_of_minimal_rcu_full/Parameter/control/enable_ffwd_vel ==
  Controller type : Constant  Value=controller_type  OutDataTypeStr=double
  Out1 : Outport
  wires:
  Controller type/1 -> Out1/1

== system Copy_of_minimal_rcu_full/Parameter/control/stiffness type ==
  Controller type : Constant  Value=controller_type  OutDataTypeStr=double
  Out1 : Outport
  wires:
  Controller type/1 -> Out1/1

== system Copy_of_minimal_rcu_full/Parameter/ipol/stiffness type ==
  Controller type : Constant  Value=controller_type  OutDataTypeStr=double
  Out1 : Outport
  wires:
  Controller type/1 -> Out1/1

== system Copy_of_minimal_rcu_full/Roboter+controller/State_Observer/First_order_filter1 ==
  x[n] : Inport  PortDimensions=7
  d_delta_p : Inport  Port=2  PortDimensions=7
  reset : Inport  Port=3  PortDimensions=1
  Sum5 : Sum  SaturateOnIntegerOverflow=on  InputSameDT=on  OutDataTypeStr=Inherit: Same as first input
  Unit Delay Resettable External IC : simulink/Additional Math & Discrete/Additional Discrete/Unit Delay Resettable External IC  tsamp=-1
  x_coeff : Gain  Gain=h./(h+T)  SaturateOnIntegerOverflow=on  OutDataTypeStr=Inherit: Same as input  ParamDataTypeStr=Inherit: Same as input
  y_coeff : Gain  Gain=T./(h+T)  SaturateOnIntegerOverflow=on  OutDataTypeStr=Inherit: Same as input  ParamDataTypeStr=Inherit: Same as input
  y[n] : Outport  PortDimensions=7  InitialOutput=0
  wires:
  d_delta_p/1 -> Unit Delay Resettable External IC/3
  x[n]/1 -> x_coeff/1
  y_coeff/1 -> Sum5/2
  Sum5/1 -> y[n]/1, Unit Delay Resettable External IC/1
  x_coeff/1 -> Sum5/1
  Unit Delay Resettable External IC/1 -> y_coeff/1
  reset/1 -> Unit Delay Resettable External IC/2

== system Copy_of_minimal_rcu_full/Roboter+controller/State_Observer/Impulse_Observer ==
  dq : Inport
  tau : Inport  Port=2
  G : Inport  Port=3
  C : Inport  Port=4
  M : Inport  Port=5  OutDataTypeStr=double  PortDimensions=[7 7]
  K1_beo : Inport  Port=6
  reset : Inport  Port=7
  Constant7 : Constant  Value=[0 0 0 0 0 0 0]
  First_order_filter4 : Subsystem  mask{h=sample_time_robot, T=1./( 2*pi *FIXED_FILTER_BANDWIDTH_OBSERVER)}
      mask help:
      | c1 = h/(h+T)
      | c2 = T/(h+T)
      | h - sampling time
      | T =1/(2*pi*f) filter time constant
      | y[n] = c1*x[n] + c2*y[n-1]
  Product : Product  RndMeth=Zero
  Reshape1 : Reshape
  Subsystem1 : Subsystem
  r : Outport
  r_unfiltered : Outport  Port=2
  p : Outport  Port=3  OutDataTypeStr=double  PortDimensions=[7 1]
  p_hat : Outport  Port=4  OutDataTypeStr=double  PortDimensions=7
  beta : Outport  Port=5  OutDataTypeStr=double  PortDimensions=7
  dM : Outport  Port=6  OutDataTypeStr=double  PortDimensions=[7 7]
  dMq : Outport  Port=7  OutDataTypeStr=double  PortDimensions=7
  n : Outport  Port=8  OutDataTypeStr=double  PortDimensions=7
  wires:
  C/1 -> Subsystem1/5(C)
  G/1 -> Subsystem1/6(G)
  Subsystem1/5(delta_p) -> Reshape1/1
  Subsystem1/7(p) -> p/1
  Subsystem1/6(p_hat) -> p_hat/1
  dq/1 -> Subsystem1/3(dq)
  Subsystem1/4("n ") -> n/1
  Subsystem1/3(dMdq) -> dMq/1
  Subsystem1/2(dM) -> dM/1
  Subsystem1/1(beta) -> beta/1
  K1_beo/1 -> Product/2
  tau/1 -> Subsystem1/2(tau)
  M/1 -> Subsystem1/1(M)
  Constant7/1 -> First_order_filter4/2(d_delta_p)
  reset/1 -> Subsystem1/7(reset), First_order_filter4/3(d_delta_p1)
  Product/1 -> First_order_filter4/1(x[n]), r_unfiltered/1
  First_order_filter4/1(y[n]) -> Subsystem1/4(r), r/1
  Reshape1/1 -> Product/1

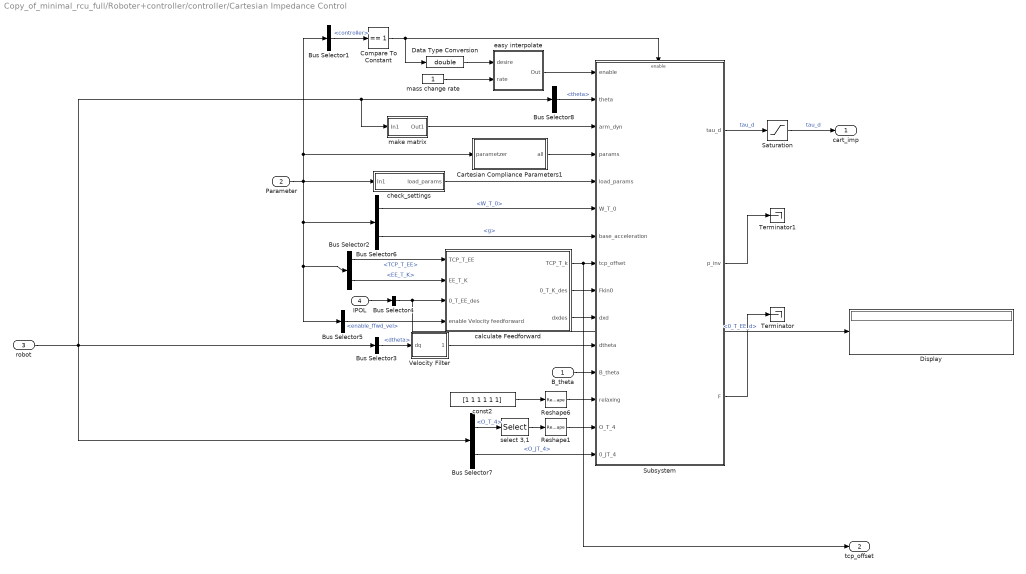
== system Copy_of_minimal_rcu_full/Roboter+controller/controller/Cartesian Impedance Control ==
  B_theta : Inport
  Parameter : Inport  Port=2
  robot : Inport  Port=3
  IPOL : Inport  Port=4
  Bus Selector1 : BusSelector  OutputSignals=controller
  Bus Selector2 : BusSelector  OutputSignals=TCP_T_EE,EE_T_K
  Bus Selector3 : BusSelector  OutputSignals=dtheta
  Bus Selector4 : BusSelector  OutputSignals=0_T_EE_d
  Bus Selector5 : BusSelector  OutputSignals=enable_ffwd_vel
  Bus Selector6 : BusSelector  OutputSignals=W_T_0,g
  Bus Selector7 : BusSelector  OutputSignals=Transform_q.O_T_4,zero_jacobians.O_JT_4
  Bus Selector8 : BusSelector  OutputSignals=theta
  Cartesian Compliance Parameters1 : Subsystem
  Compare To Constant : simulink/Logic and Bit Operations/Compare To Constant  relop===  const=1  OutDataTypeStr=uint8  ZeroCross=off
  Data Type Conversion : DataTypeConversion  OutDataTypeStr=double
  Display : Display
  Reshape1 : Reshape  OutputDimensions=[7,6]
  Reshape6 : Reshape  OutputDimensions=[7,6]
  Saturation : Saturate  UpperLimit=tau_max  LowerLimit=-tau_max
  Subsystem : Subsystem
  Terminator : Terminator
  Terminator1 : Terminator
  Velocity Filter : Subsystem
  calculate Feedforward : Subsystem
  check_settings : Subsystem
  const2 : Constant  Value=[1 1 1 1 1 1]  VectorParams1D=off
  easy interpolate : Subsystem
  make matrix : Subsystem
  mass change rate : Constant
  select 3,1 : Selector  NumberOfDimensions=2  InputPortWidth=3  IndexOptions=Index vector (dialog),Index vector (dialog)  Indices=[1:3],[1:4]  OutputSizes=1,1
  cart_imp : Outport
  tcp_offset : Outport  Port=2
  wires:
  Data Type Conversion/1 -> easy interpolate/1(desire)
  Velocity Filter/1(dq_filt) -> Subsystem/11(dtheta)
  Bus Selector3/1 -> Velocity Filter/1(dq)  "<dtheta>"
  robot/1 -> Bus Selector3/1, Bus Selector8/1, make matrix/1(In1), Bus Selector7/1
  make matrix/1(Out1) -> Subsystem/3(arm_dyn)
  Saturation/1 -> cart_imp/1  "tau_d"
  check_settings/1(load_params) -> Subsystem/5(load_params)
  Parameter/1 -> Bus Selector6/1, Bus Selector2/1, Bus Selector5/1, check_settings/1(In1), Bus Selector1/1, Cartesian Compliance Parameters1/1(parametzer)
  Cartesian Compliance Parameters1/1(all) -> Subsystem/4(params)
  Compare To Constant/1 -> Data Type Conversion/1, Subsystem/Enable
  B_theta/1 -> Subsystem/12(B_theta)
  Subsystem/1(tau_d) -> Saturation/1  "tau_d"
  const2/1 -> Reshape6/1
  Reshape6/1 -> Subsystem/13(relaxing)
  calculate Feedforward/1(TCP_T_k) -> tcp_offset/1, Subsystem/8(tcp_offset)
  calculate Feedforward/3(dxdes) -> Subsystem/10(dxd)
  Bus Selector7/1 -> select 3,1/1  "<O_T_4>"
  Bus Selector8/1 -> Subsystem/2(theta)  "<theta>"
  Bus Selector1/1 -> Compare To Constant/1  "<controller>"
  mass change rate/1 -> easy interpolate/2(rate)
  Bus Selector7/2 -> Subsystem/15(0_JT_4)  "<O_JT_4>"
  easy interpolate/1(Out) -> Subsystem/1(enable)
  Subsystem/3(F) -> Terminator/1
  Bus Selector2/1 -> calculate Feedforward/1(TCP_T_EE)  "<TCP_T_EE>"
  Bus Selector2/2 -> calculate Feedforward/2(EE_T_K)  "<EE_T_K>"
  Bus Selector6/1 -> Subsystem/6(W_T_0)  "<W_T_0>"
  Bus Selector6/2 -> Subsystem/7(base_acceleration)  "<g>"
  IPOL/1 -> Bus Selector4/1
  Bus Selector4/1 -> calculate Feedforward/3(0_T_EE_des), Display/1  "<0_T_EE_d>"
  Subsystem/2(p_inv) -> Terminator1/1
  Bus Selector5/1 -> calculate Feedforward/4(enable Velocity feedforward)  "<enable_ffwd_vel>"
  Reshape1/1 -> Subsystem/14(O_T_4)
  select 3,1/1 -> Reshape1/1
  calculate Feedforward/2(0_T_K_des) -> Subsystem/9(Fkin0)

== system Copy_of_minimal_rcu_full/Roboter+controller/controller/Joint Impedance ==
  B_theta : Inport
  parameters : Inport  Port=2
  robot : Inport  Port=3
  ipol : Inport  Port=4
  Bus Selector1 : BusSelector  OutputSignals=enable_ffwd_vel,enable_ffwd_acc
  Bus Selector2 : BusSelector  OutputSignals=K_theta,D_theta
  Bus Selector3 : BusSelector  OutputSignals=dynamics_q.Mass,dynamics_q.G
  Bus Selector4 : BusSelector  OutputSignals=theta
  Bus Selector5 : BusSelector  OutputSignals=controller
  Bus Selector6 : BusSelector  OutputSignals=theta_d,dtheta_d,ddtheta_d
  Compare To Constant : simulink/Logic and Bit Operations/Compare To Constant  relop===  const=2  OutDataTypeStr=uint8  ZeroCross=off
  JOINT_IMPEDANCE_CONTROL : Subsystem
  Joint Compliance Parameters : Subsystem
  Saturation : Saturate  UpperLimit=tau_max  LowerLimit=-tau_max
  Velocity Filter : Subsystem
  tau_d : Outport
  wires:
  Joint Compliance Parameters/1(all) -> JOINT_IMPEDANCE_CONTROL/7(joint_comp_params)
  Bus Selector3/1 -> JOINT_IMPEDANCE_CONTROL/8(M(theta))  "<Mass>"
  Bus Selector3/2 -> JOINT_IMPEDANCE_CONTROL/9(g(theta))  "<G>"
  Compare To Constant/1 -> JOINT_IMPEDANCE_CONTROL/Enable
  Saturation/1 -> tau_d/1  "tau_d"
  Velocity Filter/1(dq) -> JOINT_IMPEDANCE_CONTROL/10(dtheta)
  Bus Selector2/1 -> Joint Compliance Parameters/1(K_theta)  "<K_theta>"
  Bus Selector2/2 -> Joint Compliance Parameters/2(D_theta)  "<D_theta>"
  B_theta/1 -> JOINT_IMPEDANCE_CONTROL/11(B_theta)
  JOINT_IMPEDANCE_CONTROL/1(tau_d) -> Saturation/1  "tau_d"
  Bus Selector1/1 -> JOINT_IMPEDANCE_CONTROL/5(enable FFWD_vel)  "<enable_ffwd_vel>"
  Bus Selector1/2 -> JOINT_IMPEDANCE_CONTROL/6(enable FFWD_acc)  "<enable_ffwd_acc>"
  parameters/1 -> Bus Selector1/1, Bus Selector2/1, Bus Selector5/1
  robot/1 -> Bus Selector4/1, Bus Selector3/1
  Bus Selector4/1 -> Velocity Filter/1(q), JOINT_IMPEDANCE_CONTROL/1(theta)  "<theta>"
  Bus Selector5/1 -> Compare To Constant/1  "<controller>"
  ipol/1 -> Bus Selector6/1
  Bus Selector6/1 -> JOINT_IMPEDANCE_CONTROL/2(theta_d)  "<theta_d>"
  Bus Selector6/2 -> JOINT_IMPEDANCE_CONTROL/3(dtheta_d)  "<dtheta_d>"
  Bus Selector6/3 -> JOINT_IMPEDANCE_CONTROL/4(ddtheta_d)  "<ddtheta_d>"

== system Copy_of_minimal_rcu_full/Roboter+controller/controller/gains_selector ==
  controller : Inport
  Embedded MATLAB Function : MATLAB Function  TreatAsAtomicUnit=on
  Index Vector : MultiPortSwitch  Inputs=2
  Index Vector1 : MultiPortSwitch  Inputs=2
  K_imp : Subsystem
  K_imp_joint : Subsystem
  gains : Outport
  B_theta : Outport  Port=2
  wires:
  K_imp/2(K) -> Index Vector/2
  Index Vector/1 -> gains/1
  controller/1 -> Index Vector1/1, Index Vector/1
  K_imp_joint/2(K) -> Index Vector/3
  Index Vector1/1 -> Embedded MATLAB Function/1(KT)
  K_imp/1(K_T) -> Index Vector1/2
  K_imp_joint/1(K_T) -> Index Vector1/3
  Embedded MATLAB Function/1(B_theta_out) -> B_theta/1

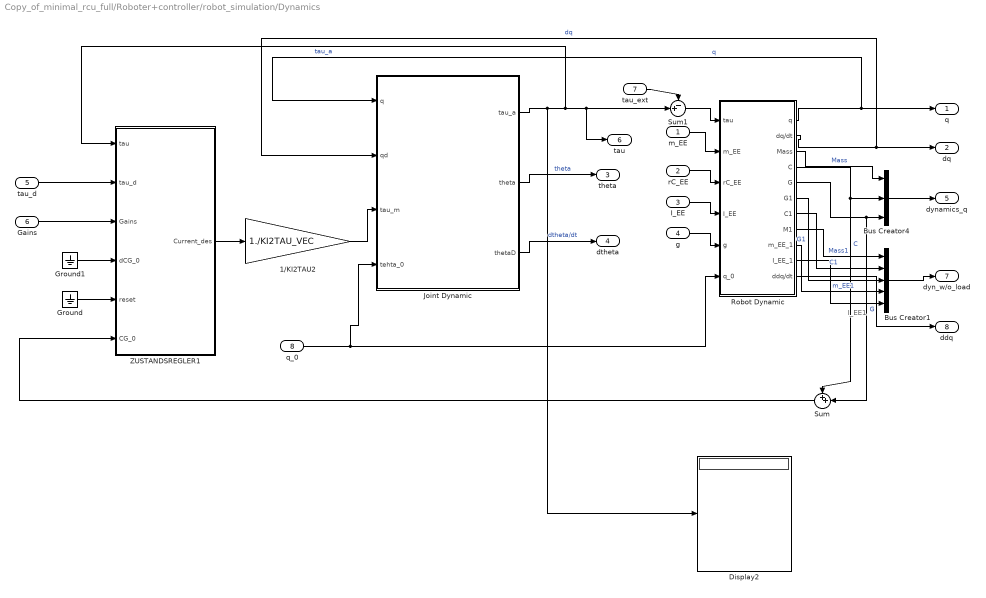
== system Copy_of_minimal_rcu_full/Roboter+controller/robot_simulation/Dynamics ==
  note: I_EE1
  m_EE : Inport
  rC_EE : Inport  Port=2
  I_EE : Inport  Port=3
  g : Inport  Port=4
  tau_d : Inport  Port=5
  Gains : Inport  Port=6
  tau_ext : Inport  Port=7
  q_0 : Inport  Port=8
  1/KI2TAU2 : Gain  Gain=1./KI2TAU_VEC  SaturateOnIntegerOverflow=on  OutDataTypeStr=Inherit: Same as input  ParamDataTypeStr=Inherit: Same as input
  Bus Creator1 : BusCreator  Inputs=5
  Bus Creator4 : BusCreator  Inputs=3
  Display2 : Display
  Ground : Ground
  Ground1 : Ground
  Joint Dynamic : Subsystem  AncestorBlock=lwr_dynamics/Dynamics/Joint Dynamic
      mask Display:
      | image(imread('lbrjoint.jpg'))
      | port_label('input', 1, 'q')
      | port_label('input', 2, 'dq/dt')
      | port_label('input', 3, 'tau_m')
      | port_label('output', 1, 'tau_a')
      | port_label('output', 2, 'theta')
      | port_label('output', 3, 'dtheta/dt')
      | port_label('output', 4, 'tau')
  Robot Dynamic : Subsystem
  Sum : Sum  Inputs=++|
  Sum1 : Sum  Inputs=-+|
  ZUSTANDSREGLER1 : Subsystem
  q : Outport
  dq : Outport  Port=2
  theta : Outport  Port=3
  dtheta : Outport  Port=4
  dynamics_q : Outport  Port=5
  tau : Outport  Port=6
  dyn_w/o_load : Outport  Port=7
  ddq : Outport  Port=8
  wires:
  Robot Dynamic/2(dq/dt) -> Joint Dynamic/2(qd), dq/1  "dq"
  Robot Dynamic/1(q) -> Joint Dynamic/1(q), q/1  "q"
  g/1 -> Robot Dynamic/5(g)
  I_EE/1 -> Robot Dynamic/4(I_EE)
  rC_EE/1 -> Robot Dynamic/3(rC_EE)
  m_EE/1 -> Robot Dynamic/2(m_EE)
  Joint Dynamic/1(tau_a) -> Display2/1, ZUSTANDSREGLER1/1(tau), tau/1, Sum1/2  "tau_a"
  Joint Dynamic/2(theta) -> theta/1  "theta"
  Joint Dynamic/3(thetaD) -> dtheta/1  "dtheta/dt"
  ZUSTANDSREGLER1/1(Current_des) -> 1/KI2TAU2/1
  tau_d/1 -> ZUSTANDSREGLER1/2(tau_d)
  1/KI2TAU2/1 -> Joint Dynamic/3(tau_m)
  Gains/1 -> ZUSTANDSREGLER1/3(Gains)
  Ground/1 -> ZUSTANDSREGLER1/5(reset)
  Robot Dynamic/3(Mass) -> Bus Creator4/1  "Mass"
  Robot Dynamic/4(C) -> Sum/1, Bus Creator4/2  "C"
  Robot Dynamic/5(G) -> Sum/2, Bus Creator4/3  "G"
  Bus Creator4/1 -> dynamics_q/1
  Ground1/1 -> ZUSTANDSREGLER1/4(dCG_0)
  Sum/1 -> ZUSTANDSREGLER1/6(CG_0)
  Sum1/1 -> Robot Dynamic/1(tau)
  tau_ext/1 -> Sum1/1
  q_0/1 -> Joint Dynamic/4(tehta_0), Robot Dynamic/6(q_0)
  Bus Creator1/1 -> dyn_w/o_load/1
  Robot Dynamic/6(G1) -> Bus Creator1/3  "G1"
  Robot Dynamic/8(M1) -> Bus Creator1/1  "Mass1"
  Robot Dynamic/7(C1) -> Bus Creator1/2  "C1"
  Robot Dynamic/9(m_EE_1) -> Bus Creator1/4  "m_EE1"
  Robot Dynamic/10(I_EE_1) -> Bus Creator1/5
  Robot Dynamic/11(ddq/dt) -> ddq/1

== system Copy_of_minimal_rcu_full/Roboter+controller/robot_simulation/model ==
  q : Inport
  TCP_T_EE : Inport  Port=2
  theta : Inport  Port=3
  Body Jacobians : Subsystem
  Jacobians to Zero : Subsystem
  forward_kin_q : Subsystem
  forward_kin_q1 : Subsystem
  body_jacobians : Outport
  zero_jacobians : Outport  Port=2
  Transforms_q : Outport  Port=3
  Transforms_theta : Outport  Port=4
  wires:
  q/1 -> Body Jacobians/1(q), Jacobians to Zero/1(q), forward_kin_q/1(q)
  Body Jacobians/1(jacobians wrt body) -> body_jacobians/1
  Jacobians to Zero/1(jacobians_wrt_zero) -> zero_jacobians/1
  forward_kin_q/1(fkin_q) -> Transforms_q/1
  TCP_T_EE/1 -> Body Jacobians/2(TCP_T_EE), Jacobians to Zero/2(TCP_T_EE), forward_kin_q/2(TCP_T_EE), forward_kin_q1/2(TCP_T_EE)
  theta/1 -> forward_kin_q1/1(q)
  forward_kin_q1/1(fkin_q) -> Transforms_theta/1

== system Copy_of_minimal_rcu_full/Ipol/joint_ipol_5th_traj_scaling/Subsystem/Cartesian_ipol1 ==
  t : Inport
  s0 : Inport  Port=2
  v0 : Inport  Port=3
  sf : Inport  Port=4
  vm : Inport  Port=5
  am : Inport  Port=6
  Enable : EnablePort
  translation : Subsystem
  qd : Outport
  ipol_finished : Outport  Port=2
  dqd : Outport  Port=3
  wires:
  translation/3(dqd) -> dqd/1
  translation/1(q_d) -> qd/1
  am/1 -> translation/6(ddq_max)
  vm/1 -> translation/5(dq_max)
  sf/1 -> translation/4(q_2)
  s0/1 -> translation/2(q_1)  "s0"
  translation/2(ipol_finnished) -> ipol_finished/1
  v0/1 -> translation/3(dq_1)
  t/1 -> translation/1(t)

== system Copy_of_minimal_rcu_full/Ipol/joint_ipol_5th_traj_scaling/Subsystem/time_generator and resets ==
  note: t-t0
  note: time t
  start : Inport
  reset : Inport  Port=2
  delta_t : Inport  Port=3
  Data Type Conversion : DataTypeConversion  OutDataTypeStr=double
  Product : Product  Inputs=3  RndMeth=Zero
  Saturation : Saturate  UpperLimit=inf  LowerLimit=0
  Subtract1 : Sum  Inputs=+-
  Subtract3 : Sum
  Triggered Subsystem : Subsystem  TreatAsAtomicUnit=on
  Unit Delay Resettable : simulink/Additional Math & Discrete/Additional Discrete/Unit Delay Resettable  vinit=0.0  tsamp=-1
  delta_time : Constant  Value=sample_time_model
  time : Outport
  wires:
  Data Type Conversion/1 -> Unit Delay Resettable/2
  start/1 -> Product/1, Triggered Subsystem/Trigger
  Subtract1/1 -> time/1
  Triggered Subsystem/1(t0) -> Subtract1/2
  delta_time/1 -> Product/2
  Product/1 -> Subtract3/1
  Unit Delay Resettable/1 -> Subtract3/2, Subtract1/1, Triggered Subsystem/1(t)
  Subtract3/1 -> Saturation/1
  reset/1 -> Data Type Conversion/1
  delta_t/1 -> Product/3
  Saturation/1 -> Unit Delay Resettable/1

== system Copy_of_minimal_rcu_full/Roboter+controller/State_Observer/Impulse_Observer/First_order_filter4 ==
  x[n] : Inport  PortDimensions=7
  d_delta_p : Inport  Port=2  PortDimensions=7
  d_delta_p1 : Inport  Port=3  PortDimensions=1
  Sum5 : Sum  SaturateOnIntegerOverflow=on  InputSameDT=on  OutDataTypeStr=Inherit: Same as first input
  Unit Delay Resettable External IC : simulink/Additional Math & Discrete/Additional Discrete/Unit Delay Resettable External IC  tsamp=-1
  x_coeff : Gain  Gain=h./(h+T)  SaturateOnIntegerOverflow=on  OutDataTypeStr=Inherit: Same as input  ParamDataTypeStr=Inherit: Same as input
  y_coeff : Gain  Gain=T./(h+T)  SaturateOnIntegerOverflow=on  OutDataTypeStr=Inherit: Same as input  ParamDataTypeStr=Inherit: Same as input
  y[n] : Outport  PortDimensions=7  InitialOutput=0
  wires:
  d_delta_p/1 -> Unit Delay Resettable External IC/3
  x[n]/1 -> x_coeff/1
  y_coeff/1 -> Sum5/2
  Sum5/1 -> y[n]/1, Unit Delay Resettable External IC/1
  x_coeff/1 -> Sum5/1
  Unit Delay Resettable External IC/1 -> y_coeff/1
  d_delta_p1/1 -> Unit Delay Resettable External IC/2

== system Copy_of_minimal_rcu_full/Roboter+controller/State_Observer/Impulse_Observer/Subsystem1 ==
  note: beta
  note: r=tau_ext_hat
  note: p_hat
  note: dp_hat
  M : Inport
  tau : Inport  Port=2
  dq : Inport  Port=3
  r : Inport  Port=4
  C : Inport  Port=5
  G : Inport  Port=6
  reset : Inport  Port=7
  Data Type Conversion : DataTypeConversion  OutDataTypeStr=double
  Integrator : Integrator  ExternalReset=either
  Reshape1 : Reshape  OutputDimensionality=Column vector (2-D)
  Sum3 : Sum  Inputs=+-
  Sum6 : Sum  Inputs=-|+|-
  calc_beta : Subsystem
  calc_n : Sum
  calc_p : Subsystem
  beta : Outport
  dM : Outport  Port=2
  dMdq : Outport  Port=3
  "n " : Outport  Port=4
  delta_p : Outport  Port=5
  p_hat : Outport  Port=6
  p : Outport  Port=7
  wires:
  dq/1 -> calc_p/2(dq), calc_beta/2(dq)
  Sum3/1 -> delta_p/1
  calc_beta/3(dMdq2) -> dMdq/1
  calc_beta/2(dM) -> dM/1
  r/1 -> Sum6/3
  tau/1 -> Sum6/2
  M/1 -> calc_p/1(M), calc_beta/1(M)
  G/1 -> calc_n/2
  C/1 -> calc_n/1
  calc_n/1 -> "n "/1, calc_beta/3(n)
  calc_beta/1("beta ") -> beta/1, Sum6/1
  Sum6/1 -> Integrator/1
  calc_p/1(p) -> p/1, Sum3/2
  Integrator/1 -> p_hat/1, Reshape1/1
  reset/1 -> Data Type Conversion/1
  Data Type Conversion/1 -> Integrator/2
  Reshape1/1 -> Sum3/1

== system Copy_of_minimal_rcu_full/Roboter+controller/controller/Cartesian Impedance Control/Cartesian Compliance Parameters1 ==
  parametzer : Inport
  Bus Selector2 : BusSelector  OutputSignals=K_x,D_x,K_NS,Xi_NS,W_NS_dir
  Constant : Constant
  Iterations : Constant  Value=5  OutDataTypeStr=double
  Mux1 : Mux  Inputs=11
  Mux3 : Mux  Inputs=2
  Product : Product  RndMeth=Zero
  Saturation : Saturate  UpperLimit=2000  LowerLimit=0
  Saturation1 : Saturate  UpperLimit=1  LowerLimit=0
  Saturation5 : Saturate  UpperLimit=200  LowerLimit=0
  Selector : Selector  InputPortWidth=6  Indices=[1:3]
  Selector1 : Selector  InputPortWidth=6  Indices=[4:6]
  damping type : Subsystem  mask{damping_type=2 ... AA}
      mask prompts: damping_type "Type"
      mask init:
      | ctrlp(1).s='Double';
      | ctrlp(2).s='AA';
      mask TypeOptions damping_type: 1 ... Double Diagonalization | 2 ... AA
      mask Display: fprintf('Ctrl = %s', ctrlp(damping_type).s)
  interpol : Subsystem
  interpol5 : Subsystem
  sing_damp : Constant  Value=25  OutDataTypeStr=double
  sing_gain : Constant  Value=5000*0  OutDataTypeStr=double
  sing_region : Constant  Value=0.05  OutDataTypeStr=double
  stiffness type : Subsystem  mask{controller_type=2 ... Spatial Stiffness}
      mask prompts: controller_type "Type"
      mask init:
      | ctrlp(1).s='Euler';
      | ctrlp(2).s='Spatial';
      mask TypeOptions controller_type: 1 ... Euler Angles | 2 ... Spatial Stiffness
      mask Display: fprintf('Ctrl = %s', ctrlp(controller_type).s)
  all : Outport
  wires:
  Saturation5/1 -> Mux3/2
  Saturation/1 -> Mux3/1
  Selector1/1 -> Saturation5/1
  Selector/1 -> Saturation/1
  Mux1/1 -> all/1
  stiffness type/1(Out1) -> Mux1/1
  Iterations/1 -> Mux1/2
  Mux3/1 -> Mux1/3
  Saturation1/1 -> Mux1/4
  Product/1 -> Selector/1, Selector1/1
  interpol5/1(Out1) -> Saturation1/1
  parametzer/1 -> Bus Selector2/1
  Bus Selector2/1 -> interpol/1(In1)  "<K_x>"
  Bus Selector2/2 -> interpol5/1(In1)  "<D_x>"
  Bus Selector2/3 -> Mux1/5  "<K_NS>"
  Bus Selector2/4 -> Mux1/6  "<Xi_NS>"
  Constant/1 -> Product/1
  interpol/1(Out1) -> Product/2
  sing_region/1 -> Mux1/8
  sing_gain/1 -> Mux1/9
  sing_damp/1 -> Mux1/10
  damping type/1(Out1) -> Mux1/11
  Bus Selector2/5 -> Mux1/7  "<W_NS_dir>"

== system Copy_of_minimal_rcu_full/Roboter+controller/controller/Cartesian Impedance Control/Subsystem ==
  enable : Inport
  theta : Inport  Port=2
  arm_dyn : Inport  Port=3
  params : Inport  Port=4
  load_params : Inport  Port=5
  W_T_0 : Inport  Port=6
  base_acceleration : Inport  Port=7
  tcp_offset : Inport  Port=8
  Fkin0 : Inport  Port=9
  dxd : Inport  Port=10
  dtheta : Inport  Port=11
  B_theta : Inport  Port=12
  relaxing : Inport  Port=13
  O_T_4 : Inport  Port=14
  0_JT_4 : Inport  Port=15
  Enable : EnablePort
  Add : Sum  Inputs=5
  Cart_Imp_Torques : Scope  NumInputPorts=5
      settings: TimeRange=2  YMin=-5~-5~-5~-5~-5  YMax=5~5~5~5~5  SaveName=ScopeData3
  Cartesian Compliance Control : Subsystem  TreatAsAtomicUnit=on
  Product : Product  RndMeth=Zero
  Product1 : Product  RndMeth=Zero
  tau_d : Outport
  p_inv : Outport  Port=2
  F : Outport  Port=3
  wires:
  enable/1 -> Product/2, Product1/1
  Cartesian Compliance Control/5(tau_stiffness) -> Product/1, Cart_Imp_Torques/3
  Product/1 -> Add/3
  Add/1 -> tau_d/1
  Cartesian Compliance Control/7(tau_damping) -> Product1/2, Cart_Imp_Torques/5
  Cartesian Compliance Control/6(tau_grav) -> Add/4, Cart_Imp_Torques/4
  Cartesian Compliance Control/4(tau_d_singularity_avoidance) -> Add/2, Cart_Imp_Torques/2  "tau_d_singu"
  Cartesian Compliance Control/3(tau_d_nullspace) -> Add/1, Cart_Imp_Torques/1  "tau_d_nullspace"
  base_acceleration/1 -> Cartesian Compliance Control/8(base_acceleration)
  dtheta/1 -> Cartesian Compliance Control/7(dtheta)
  Fkin0/1 -> Cartesian Compliance Control/6(Fkin0)
  theta/1 -> Cartesian Compliance Control/1(motor_pos)
  arm_dyn/1 -> Cartesian Compliance Control/2(arm_dyn)
  params/1 -> Cartesian Compliance Control/3(params)
  load_params/1 -> Cartesian Compliance Control/4(load_params)
  tcp_offset/1 -> Cartesian Compliance Control/5(tcp_offset)
  Cartesian Compliance Control/1(F) -> F/1
  B_theta/1 -> Cartesian Compliance Control/9(B_theta)
  relaxing/1 -> Cartesian Compliance Control/10(relaxing)
  dxd/1 -> Cartesian Compliance Control/11(dxd)
  O_T_4/1 -> Cartesian Compliance Control/12(O_T_4)
  W_T_0/1 -> Cartesian Compliance Control/13(W_T_0)
  Cartesian Compliance Control/2(p_inv) -> p_inv/1
  Product1/1 -> Add/5
  0_JT_4/1 -> Cartesian Compliance Control/14(O_JT_4)

== system Copy_of_minimal_rcu_full/Roboter+controller/controller/Cartesian Impedance Control/Velocity Filter ==
  dq : Inport
  Discrete Filter1 : Subsystem
  First_order_filter_MIMO : beasty_sfcns/Utility Functions/First_order_filter_MIMO  h=sample_time_robot  T=ones(7,1)*0.009  nr=7
  Ground : Ground
  Ground1 : Ground
  Ground2 : Ground
  Terminator : Terminator
  dq_filt : Outport  OutDataTypeStr=double  PortDimensions=7
  wires:
  dq/1 -> First_order_filter_MIMO/1
  First_order_filter_MIMO/1 -> dq_filt/1
  Discrete Filter1/1(dq_filt) -> Terminator/1
  Ground/1 -> Discrete Filter1/1(dq)
  Ground1/1 -> First_order_filter_MIMO/2
  Ground2/1 -> First_order_filter_MIMO/3
